simulink library "WBToolboxLibrary"  (R2014b)
settings: Solver=ode45  StartTime=0.0  StopTime=10.0  RelTol=1e-3
undefined symbols (not defined in the file): WBT_modelName, WBT_robotName, WBT_wbiFilename, WBT_wbiList
libraries: simulink x1
(part 2 of 2)

== system WBToolboxLibrary/wholeBodyModel/Kinematics ==
  Forward Kinematics : Subsystem  mask(Forward Kinematics){frameName='frame'}
      mask prompts: frameName "Frame name"
      mask help:
      | This block retrieves the forward kinematics of the specified frame.
      |
      | Assuming DoFs is the number of degrees of freedom of the robot:
      |
      | Input:
      | - Base pose: 4x4 matrix representing the homogenous transformation between the the base frame and the world frame.
      | - Joint configuration: Vector of size DoFs, representing the configuration of the joints.
      |
      | Output:
      | - Forward Kinematics: a 4x4 matrix representing the homogenous transformation between the specified frame and the world frame.
      |
      | Parameters:
      | - Frame name: the name of the frame. It should be specified in the URDF model.
      mask init: same as WBToolboxLibrary/wholeBodyActuators/Set References
      mask DialogControl toggleHighlighting Prompt: Toggle Config Block Highlighting
      mask DialogControl toggleHighlighting Callback:
      | [configBlock, ~] = WBToolbox.BlockInitialization(gcb, gcs);
      | 
      | try
      |     if (strcmp(get_param(configBlock,'HiliteAncestors'),'none'))
      |         hilite_system(configBlock,'find');
      |     else
      |         hilite_system(configBlock,'none');
      |     end
      | catch
      |     error('[%s:ShowConfigBlock:Callback] Failed to process config block name: %s',gcb,configBlock);
      | end
      | 
      | clear configBlock
      mask Display:
      | escapedFrameName = strrep(frameName, '_', '\_');
      | % port_label('output', 1, strcat('{}^{world} H_{',escapedFrameName,'}'), 'texmode','on')
      | 
      | port_label('input', 1, '{}^{world} H_{base}', 'texmode','on')
      | port_label('input', 2, 'Joint configuration')
      | 
      | clear escapedFrameName;
  Inverse Kinematics : Subsystem  Commented=on  InitFcn=|  mask(Forward Kinematics){baseFrame='root_link', endEffFrame='l_sole', optOption=Full Constraint (Position and Orientation), robotName=WBT_robotName, localName=WBT_modelName, wbiFile=WBT_wbiFilename, wbiList=WBT_wbiList}
      | if ~exist('WBT_robotName','var')
      |     WBT_robotName = '';
      | end
      | if ~exist('WBT_modelName','var')
      |     WBT_modelName = 'WBT_simulink';
      | end
      | if ~exist('WBT_wbiFilename','var')
      |     WBT_wbiFilename = 'yarpWholeBodyInterface.ini';
      | end
      | if ~exist('WBT_wbiList','var')
      |     WBT_wbiList = 'ROBOT_TORQUE_CONTROL_JOINTS';
      | end
      mask prompts: baseFrame "Base Frame"; endEffFrame "End Effector frame"; optOption "Optimization Option"; robotName "Robot Port Name"; localName "Model Name"; wbiFile "WBI filename"; wbiList "WBI list name"
      mask help:
      | This block retrieves the forward kinematics of the specified frame.
      |
      | Assuming DoFs is the number of degrees of freedom of the robot,
      | Input:
      | - Base pose: 4x4 matrix representing the homogenous transformation between
      |              the the base frame and the world frame.
      | - Joint configuration: Vector of size DoFs, representing the configuration
      |                        of the joints.
      |
      | Output:
      | - Forward Kinematics: a 4x4 matrix representing the homogenous transformation between
      |              the specified frame and the world frame.
      |
      | Parameters:
      | - Frame name: the name of the frame. It should be specified in the URDF model.
      |
      | - Robot Port Name: Name of the ports opened by the robot. (e.g. icub).
      |                    Set an empty string ('') to use the name specified in the
      |                    Whole Body Interface configuration file.
      | - Model Name: Prefix name of the ports opened by the underlying Whole Body Interface.
      | - WBI filename: name of the file containing the configuration of the Whole Body Interface
      | - WBI List Name: name of the list of joints used to configure the Whole Body Interface
      mask TypeOptions optOption: Full Constraint (Position and Orientation) | Position only constraint
      mask Display:
      | escapedBaseFrameName = strrep(baseFrame, '_', '\_');
      | escapedEndEffFrameName = strrep(endEffFrame, '_', '\_');
      | 
      | %port_label('output', 1, strcat('{}^{world} H_{',escapedFrameName,'}'), 'texmode','on')
      | 
      | %port_label('input', 1, '{}^{world} H_{base}', 'texmode','on')
      | %port_label('input', 2, 'Joint configuration')
      | 
      | %clear escapedFrameName;
      | 
      | 
      | % if strcmp(robotPart, 'left')
      | %     prefix = 'l';
      | % else
      | %     prefix = 'r';
      | % end
      | %
      | port_label('input', 1, strcat('{}^{',escapedBaseFrameName,'} H_{',escapedEndEffFrameName,'}^d'), 'texmode','on');
      | 
      | port_label('input', 2, '{}^{world} H_{base}', 'texmode','on')
      | port_label('input', 3, 'q_j', 'texmode','on');
      | %
      | %
      | port_label('output', 1, '{}^{world} H_{base}^d', 'texmode','on')
      | port_label('output', 2, 'q_j^d', 'texmode','on');
  Remote Inverse Kinematics : Subsystem  Commented=on  InitFcn=|  mask(Forward Kinematics){solverName='/cartesianSolver', dofs=12, optOption=Full Constraint (Position and Orientation)}
      | if ~exist('WBT_robotName','var')
      |     WBT_robotName = '';
      | end
      | if ~exist('WBT_modelName','var')
      |     WBT_modelName = 'WBT_simulink';
      | end
      | if ~exist('WBT_wbiFilename','var')
      |     WBT_wbiFilename = 'yarpWholeBodyInterface.ini';
      | end
      | if ~exist('WBT_wbiList','var')
      |     WBT_wbiList = 'ROBOT_TORQUE_CONTROL_JOINTS';
      | end
      mask prompts: solverName "Solver Name"; dofs "#Dofs"; optOption "Optimization Option"
      mask help:
      | This block retrieves the forward kinematics of the specified frame.
      |
      | Assuming DoFs is the number of degrees of freedom of the robot,
      | Input:
      | - Base pose: 4x4 matrix representing the homogenous transformation between
      |              the the base frame and the world frame.
      | - Joint configuration: Vector of size DoFs, representing the configuration
      |                        of the joints.
      |
      | Output:
      | - Forward Kinematics: a 4x4 matrix representing the homogenous transformation between
      |              the specified frame and the world frame.
      |
      | Parameters:
      | - Frame name: the name of the frame. It should be specified in the URDF model.
      |
      | - Robot Port Name: Name of the ports opened by the robot. (e.g. icub).
      |                    Set an empty string ('') to use the name specified in the
      |                    Whole Body Interface configuration file.
      | - Model Name: Prefix name of the ports opened by the underlying Whole Body Interface.
      | - WBI filename: name of the file containing the configuration of the Whole Body Interface
      | - WBI List Name: name of the list of joints used to configure the Whole Body Interface
      mask TypeOptions optOption: Full Constraint (Position and Orientation) | Position only constraint
      mask DialogControl Container8 Prompt: Block parameters
      mask Display:
      | disp(solverName)
      | 
      | 
      | 
      | % escapedBaseFrameName = strrep(baseFrame, '_', '\_');
      | % escapedEndEffFrameName = strrep(endEffFrame, '_', '\_');
      | %
      | % %port_label('output', 1, strcat('{}^{world} H_{',escapedFrameName,'}'), 'texmode','on')
      | %
      | % %port_label('input', 1, '{}^{world} H_{base}', 'texmode','on')
      | % %port_label('input', 2, 'Joint configuration')
      | %
      | % %clear escapedFrameName;
      | %
      | %
      | % % if strcmp(robotPart, 'left')
      | % %     prefix = 'l';
      | % % else
      | % %     prefix = 'r';
      | % % end
      | % %
      | 
      | port_label('input', 1, 'H^d', 'texmode','on');
      | % port_label('input', 1, strcat('{}^{',escapedBaseFrameName,'} H_{',escapedEndEffFrameName,'}^d'), 'texmode','on');
      | %
      | % port_label('input', 2, '{}^{world} H_{base}', 'texmode','on')
      | port_label('input', 2, 'q_j(0)', 'texmode','on');
      | % %
      | % %
      | % port_label('output', 1, '{}^{world} H_{base}^d', 'texmode','on')
      | port_label('output', 1, 'q_j^d', 'texmode','on');

== system WBToolboxLibrary/wholeBodyStates/Get Limits ==
  S-Function : S-Function  FunctionName=WBToolbox  Parameters='GetLimits',WBTConfigParameters,configBlockAbsName,limitsType  SFunctionDeploymentMode=off  EnableBusSupport=off
  Min : Outport
  Max : Outport  Port=2
  wires:
  S-Function/1 -> Min/1
  S-Function/2 -> Max/1

== system WBToolboxLibrary/wholeBodyStates/Get Measurement ==
  S-Function : S-Function  FunctionName=WBToolbox  Parameters='GetMeasurement',WBTConfigParameters,configBlockAbsName,measuredType  SFunctionDeploymentMode=off  EnableBusSupport=off
  Estimate : Outport
  wires:
  S-Function/1 -> Estimate/1

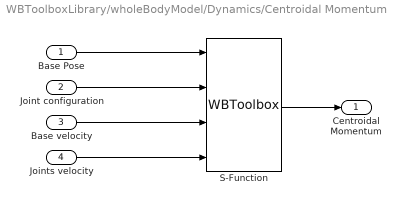
== system WBToolboxLibrary/wholeBodyModel/Dynamics/Centroidal Momentum ==
  Base Pose : Inport
  Joint configuration : Inport  Port=2
  Base velocity : Inport  Port=3
  Joints velocity : Inport  Port=4
  S-Function : S-Function  FunctionName=WBToolbox  Parameters='CentroidalMomentum',WBTConfigParameters,configBlockAbsName  SFunctionDeploymentMode=off  EnableBusSupport=off
  Centroidal Momentum : Outport
  wires:
  S-Function/1 -> Centroidal Momentum/1
  Base Pose/1 -> S-Function/1
  Joint configuration/1 -> S-Function/2
  Base velocity/1 -> S-Function/3
  Joints velocity/1 -> S-Function/4

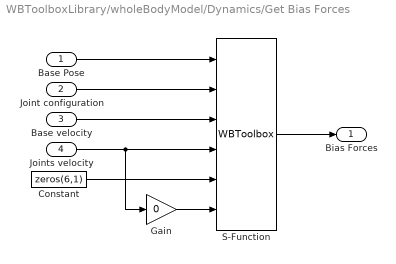
== system WBToolboxLibrary/wholeBodyModel/Dynamics/Get Bias Forces ==
  Base Pose : Inport
  Joint configuration : Inport  Port=2
  Base velocity : Inport  Port=3
  Joints velocity : Inport  Port=4
  Constant : Constant  Value=zeros(6,1)
  Gain : Gain  Gain=0
  S-Function : S-Function  FunctionName=WBToolbox  Parameters='InverseDynamics',WBTConfigParameters,configBlockAbsName  SFunctionDeploymentMode=off  EnableBusSupport=off
  Bias Forces : Outport
  wires:
  S-Function/1 -> Bias Forces/1
  Base Pose/1 -> S-Function/1
  Joint configuration/1 -> S-Function/2
  Base velocity/1 -> S-Function/3
  Joints velocity/1 -> Gain/1, S-Function/4
  Constant/1 -> S-Function/5
  Gain/1 -> S-Function/6

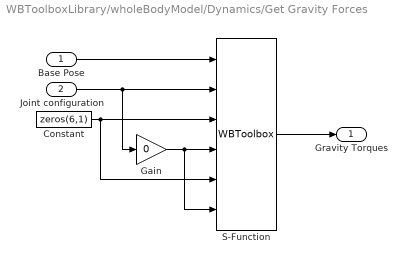
== system WBToolboxLibrary/wholeBodyModel/Dynamics/Get Gravity Forces ==
  Base Pose : Inport
  Joint configuration : Inport  Port=2
  Constant : Constant  Value=zeros(6,1)
  Gain : Gain  Gain=0
  S-Function : S-Function  FunctionName=WBToolbox  Parameters='InverseDynamics',WBTConfigParameters,configBlockAbsName  SFunctionDeploymentMode=off  EnableBusSupport=off
  Gravity Torques : Outport
  wires:
  S-Function/1 -> Gravity Torques/1
  Base Pose/1 -> S-Function/1
  Joint configuration/1 -> Gain/1, S-Function/2
  Constant/1 -> S-Function/5, S-Function/3
  Gain/1 -> S-Function/6, S-Function/4

== system WBToolboxLibrary/wholeBodyModel/Dynamics/Mass Matrix ==
  Base Pose : Inport
  Joint configuration : Inport  Port=2
  S-Function : S-Function  FunctionName=WBToolbox  Parameters='MassMatrix',WBTConfigParameters,configBlockAbsName  SFunctionDeploymentMode=off  EnableBusSupport=off
  Mass Matrix : Outport
  wires:
  S-Function/1 -> Mass Matrix/1
  Base Pose/1 -> S-Function/1
  Joint configuration/1 -> S-Function/2

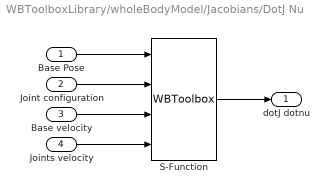
== system WBToolboxLibrary/wholeBodyModel/Jacobians/DotJ Nu ==
  Base Pose : Inport
  Joint configuration : Inport  Port=2
  Base velocity : Inport  Port=3
  Joints velocity : Inport  Port=4
  S-Function : S-Function  FunctionName=WBToolbox  Parameters='DotJNu',WBTConfigParameters,configBlockAbsName,frameName  SFunctionDeploymentMode=off  EnableBusSupport=off
  dotJ dotnu : Outport
  wires:
  Joint configuration/1 -> S-Function/2
  Base Pose/1 -> S-Function/1
  S-Function/1 -> dotJ dotnu/1
  Base velocity/1 -> S-Function/3
  Joints velocity/1 -> S-Function/4

== system WBToolboxLibrary/wholeBodyModel/Jacobians/Jacobian ==
  Base Pose : Inport
  Joint configuration : Inport  Port=2
  S-Function : S-Function  FunctionName=WBToolbox  Parameters='Jacobian',WBTConfigParameters,configBlockAbsName,frameName  SFunctionDeploymentMode=off  EnableBusSupport=off
  Forward Kinematics : Outport
  wires:
  S-Function/1 -> Forward Kinematics/1
  Base Pose/1 -> S-Function/1
  Joint configuration/1 -> S-Function/2

== system WBToolboxLibrary/wholeBodyModel/Kinematics/Forward Kinematics ==
  Base Pose : Inport
  Joint configuration : Inport  Port=2
  S-Function : S-Function  FunctionName=WBToolbox  Parameters='ForwardKinematics',WBTConfigParameters,configBlockAbsName,frameName  SFunctionDeploymentMode=off  EnableBusSupport=off
  Forward Kinematics : Outport
  wires:
  S-Function/1 -> Forward Kinematics/1
  Base Pose/1 -> S-Function/1
  Joint configuration/1 -> S-Function/2

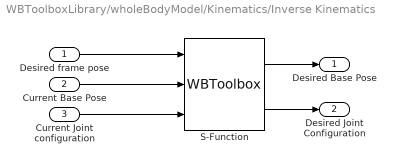
== system WBToolboxLibrary/wholeBodyModel/Kinematics/Inverse Kinematics ==
  Desired frame pose : Inport
  Current Base Pose : Inport  Port=2
  Current Joint configuration : Inport  Port=3
  S-Function : S-Function  FunctionName=WBToolbox  Parameters='InverseKinematics',robotName,localName,wbiFile,wbiList,baseFrame, endEffFrame,optOption  SFunctionDeploymentMode=off  EnableBusSupport=off
  Desired Base Pose : Outport
  Desired Joint Configuration : Outport  Port=2
  wires:
  S-Function/1 -> Desired Base Pose/1
  Current Base Pose/1 -> S-Function/2
  Current Joint configuration/1 -> S-Function/3
  Desired frame pose/1 -> S-Function/1
  S-Function/2 -> Desired Joint Configuration/1

== system WBToolboxLibrary/wholeBodyModel/Kinematics/Remote Inverse Kinematics ==
  Desired frame pose : Inport
  Current Joint configuration : Inport  Port=2
  S-Function : S-Function  FunctionName=WBToolbox  Parameters='RemoteInverseKinematics',solverName, dofs, optOption  SFunctionDeploymentMode=off  EnableBusSupport=off
  Desired Joint Configuration : Outport
  wires:
  S-Function/1 -> Desired Joint Configuration/1
  Desired frame pose/1 -> S-Function/1
  Current Joint configuration/1 -> S-Function/2

== matlab function WBToolboxLibrary/Utilities/holder /MATLAB Function ==
  data: s input; s0 output; unused input
function s0 = fcn(s, ~)
persistent state
%#codegen

if isempty(state)
    state = s;
end

s0 = state;

== matlab function WBToolboxLibrary/Utilities/DampPinv/Damped Pseudo Inverse ==
  data: mat input; DPinv output; sigma input
function DPinv  = fcn(mat,sigma)
% Economody size svd of mat
[U,S,V] = svd(mat,'econ');
% Damped version of S with sigma
S(S>sigma)=S(S>sigma)./((S(S>sigma)).^2+sigma^2);
% Damped pseudoinverse
DPinv = V*pinv(S)*U';

== matlab function WBToolboxLibrary/Utilities/TruncPinv/Truncated PseudoInverse ==
  data: mat input; TPinv output; tol input
function TPinv  = fcn(mat,tol)
%#codegen
[U,S,V] = svd(mat,'econ');
% Setting to zero value
% Setting to 1/S(i,i) singular values greater than tol
 S(S>tol)=1./S(S>tol);
 TPinv = V*pinv(S)*U';
